simulink library "csc_cmg_camera_geometry_lib"  (R2015b)
settings: Solver=ode45  SolverMode=SingleTasking  StartTime=0.0  StopTime=10.0  RelTol=1e-3
undefined symbols (not defined in the file or in its folder): cam_use_meme_flag, ini_tgt_landing_mcmf_pos
libraries: util_quat_lib x9, util_frame_rotation_lib x2, util_info_lib x1, csu_cis_camera_image_sim_lib x1, csu_kir_image_request_lib x1
settings Model: Creator=hcannon  LastModifiedBy=Mark Agbayani
settings DataIOCC: SaveFormat=Array  SignalLoggingSaveFormat=ModelDataLogs
settings OptimizationCC: BlockReduction=off  BooleanDataType=off  ExpressionDepthLimit=2147483647
settings DebuggingCC: SaveWithParameterizedLinksMsg=none  UnderspecifiedInitializationDetection=Classic  MergeDetectMultiDrivingBlocksExec=none  SignalResolutionControl=TryResolveAllWithWarning  FcnCallInpInsideContextMsg=EnableAllAsWarning  StateNameClashWarn=warning  StrictBusMsg=Warning
settings HardwareCC: ProdBitPerPointer=32  ProdLargestAtomicFloat=None  ProdIntDivRoundTo=Undefined  ProdEndianess=Unspecified  ProdWordSize=32  ProdHWDeviceType=32-bit Generic  TargetUnknown=on
settings GRTTargetCC: GeneratePreprocessorConditionals=Disable all  CombineOutputUpdateFcns=off  GRTInterface=on
settings ConfigComp: CovModelRefEnable=Off  CovSFcnEnable=off

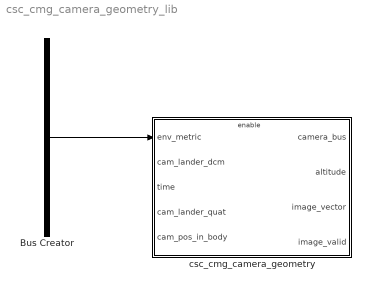
== system csc_cmg_camera_geometry_lib ==
  Bus Creator : BusCreator  Inputs=10
  csc_cmg_camera_geometry : Subsystem
  wires:
  ? -> Bus Creator/10  "grv_gravity_acc_eci"
  ? -> Bus Creator/1  "rrd_alpha_body_in_eci"
  ? -> Bus Creator/2  "rrk_rate_body_eci_body"
  ? -> Bus Creator/3  "rrk_q_body_from_eci"
  ? -> Bus Creator/4  "rrk_euler_zyx_rot_deg"
  ? -> Bus Creator/5  "rtd_acc_body_in_eci"
  ? -> Bus Creator/6  "rtk_vel_eci"
  ? -> Bus Creator/7  "rtk_pos_eci"
  ? -> Bus Creator/8
  ? -> Bus Creator/9
  Bus Creator/1 -> csc_cmg_camera_geometry/1(env_metric)

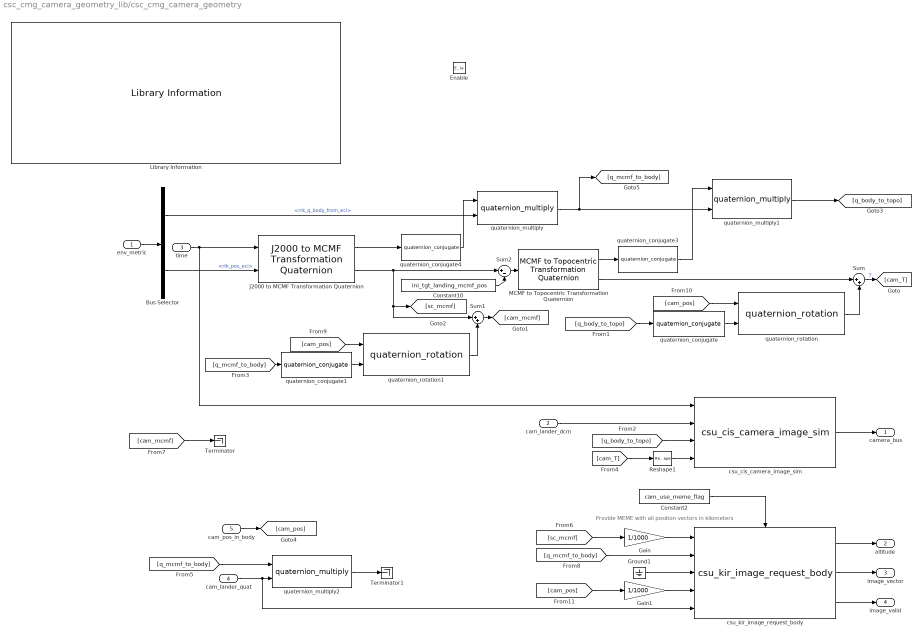
== system csc_cmg_camera_geometry_lib/csc_cmg_camera_geometry ==
  note: Provide MEME with all position vectors in kilometers
  env_metric : Inport
  cam_lander_dcm : Inport  Port=2
  time : Inport  Port=3
  cam_lander_quat : Inport  Port=4
  cam_pos_in_body : Inport  Port=5
  Enable : EnablePort
  Bus Selector : BusSelector  OutputSignals=lander_state_bus.rrk_q_body_from_eci,lander_state_bus.rtk_pos_eci
  Constant10 : Constant  Value=ini_tgt_landing_mcmf_pos
  Constant2 : Constant  Value=cam_use_meme_flag
  Gain : Gain  Gain=1/1000
  Gain1 : Gain  Gain=1/1000
  Ground1 : Ground
  J2000 to MCMF Transformation Quaternion : util_frame_rotation_lib/J2000 to MCMF  Transformation Quaternion  SystemSampleTime=-1
  Library Information : util_info_lib/Library Information  owner='NONE'
  MCMF to Topocentric Transformation Quaternion : util_frame_rotation_lib/MCMF to Topocentric  Transformation Quaternion  SystemSampleTime=-1
  Reshape1 : Reshape  OutputDimensionality=Column vector (2-D)
  Sum : Sum  Inputs=|++
  Sum1 : Sum  Inputs=|++
  Sum2 : Sum  Inputs=|+-
  Terminator : Terminator
  Terminator1 : Terminator
  csu_cis_camera_image_sim : csu_cis_camera_image_sim_lib/csu_cis_camera_image_sim
  csu_kir_image_request_body : csu_kir_image_request_lib/csu_kir_image_request_body  size=cam_kir_image_size  intrinsics=cam_kir_intrinsics
  quaternion_conjugate{,1,3..4} (4 alike) : util_quat_lib/quaternion_conjugate  SystemSampleTime=-1
  quaternion_multiply : util_quat_lib/quaternion_multiply  SystemSampleTime=-1
  quaternion_multiply1 : util_quat_lib/quaternion_multiply  SystemSampleTime=-1
  quaternion_multiply2 : util_quat_lib/quaternion_multiply  SystemSampleTime=-1
  quaternion_rotation : util_quat_lib/quaternion_rotation  SystemSampleTime=-1
  quaternion_rotation1 : util_quat_lib/quaternion_rotation  SystemSampleTime=-1
  camera_bus : Outport
  altitude : Outport  Port=2
  image_vector : Outport  Port=3
  image_valid : Outport  Port=4
  wires:
  Gain1/1 -> csu_kir_image_request_body/4
  [cam_pos] -> Gain1/1
  cam_pos_in_body/1 -> [cam_pos]
  [cam_mcmf] -> Terminator/1
  Constant2/1 -> csu_kir_image_request_body/Enable
  Reshape1/1 -> csu_cis_camera_image_sim/4
  csu_cis_camera_image_sim/1 -> camera_bus/1
  [q_body_to_topo] -> csu_cis_camera_image_sim/3
  cam_lander_dcm/1 -> csu_cis_camera_image_sim/2
  Sum2/1 -> MCMF to Topocentric Transformation Quaternion/1
  J2000 to MCMF Transformation Quaternion/2 -> Sum1/1, [sc_mcmf], Sum2/1
  Constant10/1 -> Sum2/2
  csu_kir_image_request_body/2 -> image_vector/1
  Ground1/1 -> csu_kir_image_request_body/3
  [sc_mcmf] -> Gain/1
  [q_mcmf_to_body] -> quaternion_multiply2/1
  Sum1/1 -> [cam_mcmf]
  quaternion_rotation1/1 -> Sum1/2
  [q_mcmf_to_body] -> quaternion_conjugate1/1
  quaternion_conjugate1/1 -> quaternion_rotation1/2
  [cam_pos] -> quaternion_rotation1/1
  time/1 -> J2000 to MCMF Transformation Quaternion/1, csu_cis_camera_image_sim/1
  [cam_T] -> Reshape1/1
  J2000 to MCMF Transformation Quaternion/1 -> quaternion_conjugate4/1
  quaternion_conjugate4/1 -> quaternion_multiply/1
  Bus Selector/1 -> quaternion_multiply/2  "<rrk_q_body_from_eci>"
  quaternion_multiply/1 -> quaternion_multiply1/2, [q_mcmf_to_body]
  quaternion_conjugate3/1 -> quaternion_multiply1/1
  MCMF to Topocentric Transformation Quaternion/1 -> quaternion_conjugate3/1
  quaternion_conjugate/1 -> quaternion_rotation/2
  quaternion_multiply1/1 -> [q_body_to_topo]
  MCMF to Topocentric Transformation Quaternion/2 -> Sum/1
  env_metric/1 -> Bus Selector/1
  Bus Selector/2 -> J2000 to MCMF Transformation Quaternion/2  "<rtk_pos_eci>"
  [q_body_to_topo] -> quaternion_conjugate/1
  [cam_pos] -> quaternion_rotation/1
  quaternion_rotation/1 -> Sum/2
  Sum/1 -> [cam_T]  "T"
  Gain/1 -> csu_kir_image_request_body/1
  cam_lander_quat/1 -> csu_kir_image_request_body/5, quaternion_multiply2/2
  [q_mcmf_to_body] -> csu_kir_image_request_body/2
  quaternion_multiply2/1 -> Terminator1/1
  csu_kir_image_request_body/3 -> image_valid/1
  csu_kir_image_request_body/1 -> altitude/1
